simulink model "SimulationModel"  (R2015b)
settings: Solver=ode3  SolverMode=SingleTasking  StartTime=0.0  StopTime=inf  RelTol=1e-3
PreLoadFcn:
  | addLibrariesInPath('sim')
PostLoadFcn:
  | loadRobotParameters
StartFcn:
  | simApp = SimDisplay.getInstance;
  | simApp.reset;
  | simApp.TrackView.setup(double(SitesPositions), ObstaclesPositions,ObstaclesVertices,ObstaclesEdges);
undefined symbols (not defined in the file): AngularSpeed, AxleLength, do_one_run, EncL_init, EncR_init, EncRes, lcam, motorL, motorR, motorX, ObstaclesEdges, ObstaclesVertices, pcam, SitesPositions, startPos, TauMotor, theta0, Ts, WheelRadius
libraries: simulink x2, realtime_pacer_lib x1, cstblocks x1, simulink_extras x1
(part 2 of 2)

== matlab function SimulationModel/RobotModel/Robot/Sensors Camera_Distance/Camera/relative_to_targets ==
  data: robotPos input size=[1 2]; robotTheta input size=1; dist output; bear output; SitesPositions parameter single; ObstaclesVertices parameter; ObstaclesEdges parameter; pcam parameter; lcam parameter
 function [dist,bear] = targets(robotPos,robotTheta,SitesPositions,ObstaclesVertices, ObstaclesEdges, pcam,lcam)
%#codegen
%% TARGETS Returns distance and bearing for each target relative tos robot
%
% Distances and positions are in cm
% Angles are in degrees
%
% Inputs
%   - hCam: Cam height (from ground)
%   - targetsPos: Position of targets (X,Y)
%   - robotPos: Robot position (X,Y)
%   - robotTheta: Robot angle
%
% Outputs
%   - dist (array nx1 with n=nb targets): Distances for each target,
%       if a target cannot be seen by the camera associated distance
%       is equal to -1
%   - bearing (array nx1 with n=nb targets): Angles for each target,
%       if a target cannot be seen by the camera associated angle is
%       equal to -1
%

% Get camera field of vision
% [pcam,lcam]=camera(hCam);
% betaCam = 21 ;
% etaCam = 27 ;
% [pcam, lcam] = cameraAnalytic(hCam,90-alphaCam, betaCam, etaCam);

% Convert target position to robot reference
[x,y] = world2robot(robotPos(1),robotPos(2),robotTheta,SitesPositions(:,1),SitesPositions(:,2));

% Convert Obstacles positions to robot reference
[vx,vy] = world2robot(robotPos(1),robotPos(2),robotTheta,ObstaclesVertices(:,1),ObstaclesVertices(:,2));

% Get left and right detector indicators
%[leftFlag, rightFlag] = isThereSomething(vx, vy, obstaclesEdges);

% Get distance and bearing for each point relative to robot
[distance,bearing] = isincamera(pcam,lcam,x,y,vx,vy,ObstaclesEdges);

% sort by descending order and return 6 elements
[distance,idxsort] = sort(distance,'descend');
bearing = bearing(idxsort);
if length(distance)<6
    dist = [distance;zeros(6-length(distance),1)];
    bear = [bearing;zeros(6-length(bearing),1)] ;
else
    dist = distance(1:6);
    bear = bearing(1:6);
end

end

function [x_new,y_new]=world2robot(x_robot,y_robot,theta_robot,x_world,y_world)
% WORLD2ROBOT Convert coordinates from world to robot
%
% Inputs
%   - x_robot: Robot X position (in world reference)
%   - y_robot: Robot Y position (in world reference)
%   - theta_robot: Robot angle  (in world reference)
%   - x_world: X value(s) to convert (in world reference)
%   - y_world: Y value(s) to convert (in world reference)
%
% Outpus
%   - x_new: Point(s) coordinate (X) in robot reference
%   - y_new: Point(s) coordinate (Y) in robot reference

% Translate coordinates reference
x_dif=x_world-x_robot;
y_dif=y_world-y_robot;

% Rotate coordinates reference
% x_new=x_dif*cosd(theta_robot)-y_dif*sind(theta_robot);
% y_new=x_dif*sind(theta_robot)+y_dif*cosd(theta_robot);
x_new = cosd(theta_robot)*x_dif + sind(theta_robot)*y_dif;
y_new = cosd(theta_robot)*y_dif - sind(theta_robot)*x_dif;
% see http://www.mathematics-online.org/inhalt/aussage/aussage444/

% TODO We have identified that the sign of converted coordinates is the
% opposite of the expected but we don't have an explanation for that
% x_new = -x_new;
% y_new = -y_new;

end

function [dist,bearing]=isincamera(p,l,x,y,vx,vy,OE)
%% ISINCAMERA Distance and angle from current robot position
%
% Inputs
%   - p (2 elements vector): Minimal and maximal depth for camera (Y axis)
%   - l (2 elements vector): Minimal and maximal width for camera (X axis)
%   - x (vector): X coordinate of point(s)
%   - y (vector): Y coordinate of point(s)
%
% Outputs
%   - dist (vector): Distance of each point from camera (robot), -1 if
%       point cannot be seen by camera.
%   - bearing (vector): Angle of each point from camera (robot), -1 if
%       point cannot be seen by camera.
%

% Calculate coefficients for lines that defines the camera field of vision
% Field vision limits in Y axis are constants (y = p(1) or y = p(2))
% c1=polyfit(p(1:2),[-l(1)/2 -l(2)/2],1);
% c2=polyfit(p(1:2),[l(1)/2 l(2)/2],1);

% To be visible a point must match all the following criterion
%   - Y >= minimal depth
%   - Y <= maximal depth
%   - X >= - (width for current Y) / 2
%   - X <=   (width for current Y) / 2
%

%isvisible = y>=p(1) & y<=p(2) & (x>=polyval(c1,y) & x<=polyval(c2,y));
% isvisible = x>=p(1) & x<=p(2) & (y>=polyval(c1,x) & y<=polyval(c2,x));

%TTx = [p(1) p(2) p(2) p(1)]' ;
%TTy = [l(1)/2 l(2)/2 -l(2)/2 -l(1)/2]' ;
%TTx = [[p(1); p(2); p(1)] [p(1); p(2); p(2)]];
%TTy = [[l(1)/2; l(2)/2; -l(1)/2] [-l(1)/2; l(2)/2; -l(2)/2]];
TTx = [p(1); p(2); p(2); p(1)];
TTy = [l(1)/2; l(2)/2; -l(2)/2; -l(1)/2];

[vpX, vpY] = CastRays(0, 0, [vx vy], OE);
vpX = vpX(2:end,:);
vpX = vpX(:);
vpY = vpY(2:end,:);
vpY = vpY(:);

%dis = simDisplay.getInstance;
%patch(vpX, vpY, zeros(size(vpX)), 'Parent', dis.TrackView.Axes);


isvisible = true(size(x));
for k=1:length(isvisible)
    isvisible(k) = any(myInpolygon(x(k), y(k), TTx, TTy)) && ...
        any(myInpolygon(x(k), y(k), vpX, vpY));
%     isvisible(k) = any(inTriangle(x(k), y(k), TTx, TTy)) &&...
%         any(inTriangle(x(k), y(k), vpX, vpY));
end

% Calculate distance and bearing for all points
dist = sqrt(x.^2 + y.^2);
% bearing = atan2d(y,x);
bearing = atan2d(x,-y)-90;

% Replace values by -1 for points that are not visible
dist(~isvisible) = 0;
bearing(~isvisible) = 0;

end

function [vpX, vpY] = CastRays(x, y, vertices, edges)
% Cast rays

vertices = [vertices zeros(length(vertices),5)];
% Compute relative cartesian coordinates
vertices(:,3) = vertices(:,1) -...
    x;

vertices(:,4) = vertices(:,2) -...
    y;


% Compute relative polar coordinates
[vertices(:,5), vertices(:,6)] =...
    cart2pol(vertices(:,3), vertices(:,4));

vertices(:,5) = mod(vertices(:,5), 2*pi);


% Sort rows by angle and get reverse permutation
[vertices, ind] = sortrows(vertices, 5);

[~, ind] = sort(ind, 'ascend');


% Modify the edges indices accordingly
edges(:,1) = ind(edges(:,1));

edges(:,2) = ind(edges(:,2));


% Ensure that the left vertex of each edge is on the left
Tdiff = vertices(edges(:,1),5) -...
    vertices(edges(:,2),5);

ind = xor(Tdiff < 0, abs(Tdiff)>pi);

edges(ind, [1 2]) =...
    edges(ind, [2 1]);

vpX = zeros(3, size(vertices,1));
vpY = zeros(3, size(vertices,1));


% Loop over each vertex and get the left vertex of the
% right triangle and the right edge of the left triangle
for ray = 1:size(vertices,1)
    
    % Find edges that cross the ray
    TdiffL = vertices(edges(:,1),5) -...
        vertices(ray,5);
    TdiffR = vertices(ray,5) -...
        vertices(edges(:,2),5);
    intersects = find(xor(TdiffL >= 0, abs(TdiffL)>pi) &...
        xor(TdiffR >= 0, abs(TdiffR)>pi));
    
    
    % Compute intersection coordinates
    [~, ~, interX, interY] = lineSegmentsIntersection(x, y, vertices(ray,1),...
        vertices(ray,2), vertices(edges(intersects,1),1),...
        vertices(edges(intersects,1),2), vertices(edges(intersects,2),1),...
        vertices(edges(intersects,2),2));
    
    
    % Sort the intersections (coordinates and index of the
    % edges) by distance to viewpoint
    [~, dist2vp] = cart2pol(interX - x, interY - y);
    
    [~,ind] = sort(dist2vp, 'ascend');
    
    intersects = intersects(ind);
    
    
    % Pick the first intersection, with the exception that it
    % must not be a right edge for the left triangle or a left
    % edge for the right triangle. Assign the result
    leftInd = find(edges(intersects,2) ~= ray, 1, 'first');
    rightInd = find(edges(intersects,1) ~= ray, 1, 'first');
    if isempty(leftInd)
        leftInd = 1;
    end
    if isempty(rightInd)
        rightInd = 1;
    end
    rightInd = rightInd(1);
    leftInd = leftInd(1);
    
    vpX(1,ray) = x;
    vpY(1,ray) = y;
    
    vpX(2,ray) = interX(ind(rightInd));
    vpY(2,ray) = interY(ind(rightInd));
    
    indBack = mod(ray-2, size(vertices,1))+1;
    vpX(3,indBack) = interX(ind(leftInd));
    vpY(3,indBack) = interY(ind(leftInd));
    
end

end

== matlab function SimulationModel/RobotModel/Robot/Sensors Camera_Distance/Camera/dist_bearing2locatedTargets ==
  data: robotPos input; dist input; locatedTargets output; bearing input; robotTheta input
function locatedTargets = fcn(robotPos, dist, bearing, robotTheta)
%#codegen

loc = dist > 0;

locatedTargetsX = zeros(size(dist));
locatedTargetsY = locatedTargetsX;

targetTheta = robotTheta + bearing(loc);

locatedTargetsX(loc) = robotPos(1) + dist(loc) .* cosd(targetTheta);
locatedTargetsY(loc) = robotPos(2) + dist(loc) .* sind(targetTheta);

locatedTargets = [locatedTargetsX, locatedTargetsY];

== stateflow chart SimulationModel/InputProcessing/ObstacleDetection ==
  state LeftSensor [parallel]
    settings: executionOrder=1
    state Obstacle
      entry:
      LeftObstacle = true;
    state Nothing
      entry:
      LeftObstacle = false;
    (default) -> LeftSensor.Nothing
    LeftSensor.Nothing -> LeftSensor.Obstacle : [Robot.ScannerStatus == EPosition.LEFT && ...
        | Robot.ScannerValues(EPosition.LEFT) > -1]
    LeftSensor.Obstacle -> LeftSensor.Nothing : [Robot.ScannerStatus == EPosition.LEFT && ...
        | Robot.ScannerValues(EPosition.LEFT) == -1]
  state RightSensor [parallel]
    settings: executionOrder=2
    state Obstacle
      entry:
      RightObstacle = true;
    state Nothing
      entry:
      RightObstacle = false;
    (default) -> RightSensor.Nothing
    RightSensor.Nothing -> RightSensor.Obstacle : [Robot.ScannerStatus == EPosition.RIGHT && ...
        | Robot.ScannerValues(EPosition.RIGHT) > -1]
    RightSensor.Obstacle -> RightSensor.Nothing : [Robot.ScannerStatus == EPosition.RIGHT && ...
        | Robot.ScannerValues(EPosition.RIGHT) == -1]
  state MiddleSensor [parallel]
    settings: executionOrder=3
    state Obstacle
      entry:
      MiddleObstacle = true;
    state Nothing
      entry:
      MiddleObstacle = false;
    (default) -> MiddleSensor.Nothing
    MiddleSensor.Nothing -> MiddleSensor.Obstacle : [Robot.ScannerStatus == EPosition.MIDDLE && ...
        | Robot.ScannerValues(EPosition.MIDDLE) > -1]
    MiddleSensor.Obstacle -> MiddleSensor.Nothing : [Robot.ScannerStatus == EPosition.MIDDLE && ...
        | Robot.ScannerValues(EPosition.MIDDLE) == -1]
  state Correction [parallel]
    settings: executionOrder=4
    (default) -> (junction 96)
    Correction -> (junction 96)
    (junction 96) -> (junction 97) [order 1] : [MiddleObstacle]
    (junction 96) -> (junction 98) [order 2]
    (junction 97) -> (junction 107) : {correction_status = EObstacles.AVOIDANCE;}
    (junction 98) -> (junction 99) [order 1] : [LeftObstacle]
    (junction 107) -> (junction 109) [order 1] : [LeftObstacle]
    (junction 98) -> (junction 100) [order 2]
    (junction 99) -> (junction 104) : {
        | correction_status = EObstacles.CORRECTION;
        | correction_sign = single(1);
        | }
    (junction 107) -> (junction 105) [order 2] : {correction_sign =single(-1);}
    (junction 109) -> (junction 116) : {correction_sign =single(1);}
    (junction 100) -> (junction 101) [order 1] : [RightObstacle]
    (junction 100) -> (junction 102) [order 2] : {correction_status = EObstacles.NONE;}
    (junction 101) -> (junction 103) : {
        | correction_status = EObstacles.CORRECTION;
        | correction_sign = single(-1);
        | }
    (junction 103) -> (junction 102)
    (junction 104) -> (junction 103)
    (junction 105) -> (junction 104)
    (junction 116) -> (junction 105)
    (junction 102) -> (junction 106)
  data: Robot input Bus: bus_Robot; correction_status output Enum: EObstacles; LeftObstacle local boolean; RightObstacle local boolean; MiddleObstacle local boolean; correction_sign output single

== stateflow chart SimulationModel/RobotModel/Controller/FeedbackController/ControllerModes ==
  state CurrentMove [parallel]
    settings: executionOrder=1
    state Normal
      entry:
      EncodersZero = Encoders;
      entry,during:
      [CurrentAngle,CurrentDistance] = CurrentMoveFcn(Encoders,EncodersZero);
    state [angle,distance] = CurrentMoveFcn(enc,zero) [function]
    (default) -> Normal
    Normal -> Normal : Reset
  state ModeControl [parallel]
    settings: executionOrder=2
    state DistanceControl
      entry:
      CurrentMove.Reset;
      ResetDistancePI;
      ResetAnglePI;
      entry,during:
      AngleError = Cmd.Angle - CurrentAngle;
      DistanceError = Cmd.Position - CurrentDistance;
    state SpeedControl
      entry:
      CurrentMove.Reset;
      ResetDistancePI;
      ResetAnglePI;
      state DistanceIntegration [parallel]
        settings: executionOrder=1
        (default) -> (junction 34) : {
            | DistanceCmd = single(0);
            | }
        DistanceIntegration -> (junction 34)
        (junction 34) -> (junction 35) [order 1] : [Cmd.Position == 0]
        (junction 34) -> (junction 36) [order 2] : {
            | DistanceCmd = ...
            | DistanceCmd + ...
            | Cmd.Position * single(Ts);
            | }
        (junction 35) -> (junction 37) : {
            | CurrentMove.Reset;
            | ResetDistancePI;
            | DistanceCmd = single(0) ;
            | }
        (junction 37) -> (junction 36)
        (junction 36) -> (junction 38)
      state AngleIntegration [parallel]
        settings: executionOrder=2
        (default) -> (junction 46) : {
            | AngleCmd = single(0);
            | }
        AngleIntegration -> (junction 46)
        (junction 46) -> (junction 52) [order 1] : [Cmd.Angle == 0]
        (junction 46) -> (junction 50) [order 2] : {
            | AngleCmd = ...
            | AngleCmd + ...
            | Cmd.Angle * single(Ts);
            | }
        (junction 52) -> (junction 49) : {
            | CurrentMove.Reset;
            | ResetAnglePI;
            | AngleCmd = single(0);
            | }
        (junction 49) -> (junction 50)
        (junction 50) -> (junction 48)
      state ErrorCalculation [parallel]
        entry,during:
        AngleError = AngleCmd - CurrentAngle;
        DistanceError = DistanceCmd - CurrentDistance;
        settings: executionOrder=3
    (default) -> (junction 73)
    (junction 73) -> (junction 72) [order 1] : [Cmd.Mode == EMode.SPEED]
    (junction 73) -> DistanceControl [order 2]
    (junction 72) -> SpeedControl
    SpeedControl -> DistanceControl : [Cmd.Mode == EMode.DISTANCE]
    DistanceControl -> SpeedControl : [Cmd.Mode == EMode.SPEED]
  data: enc function_input int32 size=2; zero function_input int32 size=2; angle function_output; distance function_output; DistanceCmd local single; AngleCmd local single; Encoders input int32 size=2; EncodersZero local int32 size=2; CurrentAngle local single; CurrentDistance local single; AngleError output single size=1; DistanceError output single size=1; Cmd input Bus: bus_Command; Ts parameter
  events: Reset local FUNCTION_CALL_EVENT; ResetAnglePI output EITHER_EDGE_EVENT; ResetDistancePI output EITHER_EDGE_EVENT
